simulink model "temp"  (R2018b)
settings: Solver=VariableStepAuto  StartTime=0.0  StopTime=10.0  RelTol=1e-3
values from neighbouring files (symbols this model uses):
  phi_init = deg2rad(0)    [Initial_posture.m]
  psi_init = deg2rad(0)    [Initial_posture.m]
  v_init = 1    [Initial_posture.m]
  xCr_init = 0    [Initial_posture.m]
  yCr_init = 0    [Initial_posture.m]
libraries: simulink x1
settings Model: Creator=Mahesh  LastModifiedBy=Mahesh

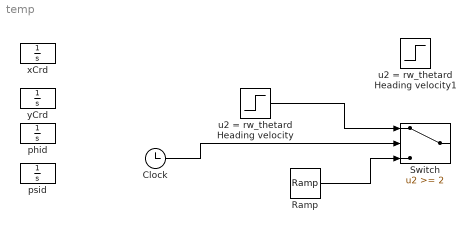
== system temp ==
  Clock : Clock
  Ramp : simulink/Sources/Ramp  slope=0.5  start=0  InitialOutput=0
  Switch : Switch  Threshold=2
  phid : Integrator  InitialCondition=phi_init
  psid : Integrator  InitialCondition=psi_init
  u2 = rw_thetard Heading velocity : Step  Time=2  SampleTime=0
  u2 = rw_thetard Heading velocity1 : Step  Time=0  After=v_init  SampleTime=0
  xCrd : Integrator  InitialCondition=xCr_init
  yCrd : Integrator  InitialCondition=yCr_init
  wires:
  Ramp/1 -> Switch/3
  u2 = rw_thetard Heading velocity/1 -> Switch/1
  Clock/1 -> Switch/2
